simulink model "scheme_robust_control"  (R2025a)
settings: Solver=ode3  StartTime=0.0  StopTime=40  FixedStep=dt  RelTol=1e-3
values from neighbouring files (symbols this model uses):
  dt = 0.01    [Planning_Adaptive_LTV.m]
  initial_positions_rad = rawJointPositions(1, :)'    [manipulator_sim.m]
  map_scale = 0.5    [Planning_Adaptive_LTV.m]
  N = numel(theta_points_rad)    [create_LPV_linearizer.m]
  waypoints = pathObj.States(:, 1:2)    [Planning_Adaptive_LTV.m]
  x0 = zeros(10, 1)    [Planning_Adaptive_LTV.m]
undefined symbols (not defined in the file or in its folder): control_params, p, X, Y, Z
libraries: sm_lib x179, nesl_utility x28, fl_lib x3, robotmaniplib x2
(part 4 of 4)

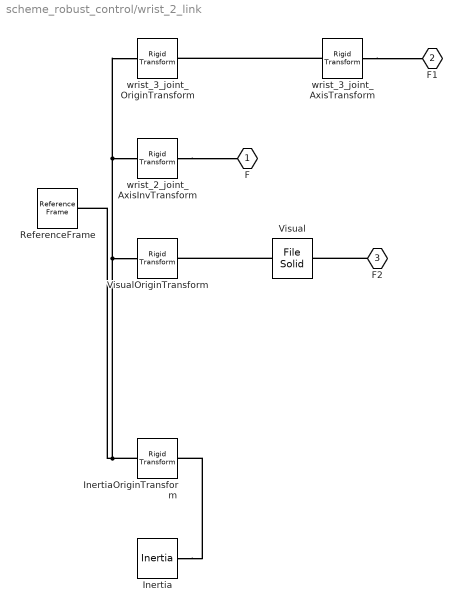
== system scheme_robust_control/wrist_2_link ==
  Inertia : sm_lib/Body Elements/Inertia  InertiaType=Custom  Mass=1.3  MassUnits=kg  CenterOfMass=[0, 0, 0]  CenterOfMassUnits=m  MomentsOfInertia=[0.00135617, 0.00096614, 0.00127827]  MomentsOfInertiaUnits=kg*m^2  ProductsOfInertia=[5.048000000000011e-05, 2.739999999999998e-06, 4.440000000000001e-06]  ProductsOfInertiaUnits=kg*m^2  GraphicType=None  MarkerShape=Inertia  MarkerSize=20  GraphicVisPropType=SimpleVisualProperties  GraphicDiffuseColor=[0.5 0.5 0.5]  GraphicOpacity=1  GraphicSpecularColor=[0.5 0.5 0.5 1.0]  GraphicAmbientColor=[0.15 0.15 0.15 1.0]  GraphicEmissiveColor=[0.0 0.0 0.0 1.0]  GraphicShininess=75
  InertiaOriginTransform : sm_lib/Frames and Transforms/Rigid Transform  RotationMethod=RotationSequence  FollAlignAxisA=+X  BaseAlignAxisA=+Y  FollAlignAxisB=+Y  BaseAlignAxisB=+Z  RotationStandardAxis=+Z  RotationAngle=0  RotationAngleUnits=deg  RotationArbitraryAxis=[0 0 1]  RotationSequenceAxes=BaseAxes  RotationSequence=XYZ  RotationSequenceAngles=[0, 0, 0]  RotationSequenceAnglesUnits=rad  RotationMatrix=[1 0 0;0 1 0;0 0 1]  Quaternion=[1 0 0 0]  TranslationMethod=Cartesian  TranslationCartesianOffset=[0, 0.01634, -0.0018]  TranslationCartesianOffsetUnits=m  TranslationStandardAxis=+Z  TranslationStandardOffset=0  TranslationStandardOffsetUnits=m  TranslationROffset=0  TranslationROffsetUnits=m  TranslationThetaOffset=0  TranslationThetaOffsetUnits=deg  TranslationZOffset=0  TranslationZOffsetUnits=m
  ReferenceFrame : sm_lib/Frames and Transforms/Reference Frame
  Visual : sm_lib/Body Elements/File Solid  ExtGeomFileName=C:\Users\chiar_zjcy1by\MATLAB Drive\FieldProject\generated\ros_packages\ur_description\meshes\ur5e\visual\wrist2.dae  UnitType=Custom  ExtGeomFileUnits=m  StepReaderType=HEX  ExportConvexHullGeometry=on  InertiaType=Custom  BasedOnType=DensityFromFile  Density=1000  DensityUnits=kg/m^3  Mass=0  MassUnits=kg  CenterOfMass=[0, 0, 0]  CenterOfMassUnits=m  MomentsOfInertia=[0, 0, 0]  MomentsOfInertiaUnits=kg*m^2  ProductsOfInertia=[0, 0, 0]  ProductsOfInertiaUnits=kg*m^2  GraphicType=FromGeometry  MarkerShape=Sphere  MarkerSize=10  GraphicVisPropType=SimpleVisualProperties  GraphicDiffuseColor=[0.5, 0.5, 0.5]  GraphicOpacity=1  GraphicSpecularColor=[0.5 0.5 0.5 1.0]  GraphicAmbientColor=[0.15 0.15 0.15 1.0]  GraphicEmissiveColor=[0.0 0.0 0.0 1.0]  GraphicShininess=75  DoExposeReferenceFrame=on  SerializedFrames=<Frames/>
  VisualOriginTransform : sm_lib/Frames and Transforms/Rigid Transform  RotationMethod=RotationSequence  FollAlignAxisA=+X  BaseAlignAxisA=+Y  FollAlignAxisB=+Y  BaseAlignAxisB=+Z  RotationStandardAxis=+Z  RotationAngle=0  RotationAngleUnits=deg  RotationArbitraryAxis=[0 0 1]  RotationSequenceAxes=BaseAxes  RotationSequence=XYZ  RotationSequenceAngles=[0, 0, 0]  RotationSequenceAnglesUnits=rad  RotationMatrix=[1 0 0;0 1 0;0 0 1]  Quaternion=[1 0 0 0]  TranslationMethod=Cartesian  TranslationCartesianOffset=[0, 0, -0.0997]  TranslationCartesianOffsetUnits=m  TranslationStandardAxis=+Z  TranslationStandardOffset=0  TranslationStandardOffsetUnits=m  TranslationROffset=0  TranslationROffsetUnits=m  TranslationThetaOffset=0  TranslationThetaOffsetUnits=deg  TranslationZOffset=0  TranslationZOffsetUnits=m
  wrist_2_joint_AxisInvTransform : sm_lib/Frames and Transforms/Rigid Transform  RotationMethod=ArbitraryAxis  FollAlignAxisA=+X  BaseAlignAxisA=+Y  FollAlignAxisB=+Y  BaseAlignAxisB=+Z  RotationStandardAxis=+Z  RotationAngle=0  RotationAngleUnits=rad  RotationArbitraryAxis=[1, 0, 0]  RotationSequenceAxes=FollowerAxes  RotationSequence=XYX  RotationSequenceAngles=[0 0 0]  RotationSequenceAnglesUnits=deg  RotationMatrix=[1 0 0;0 1 0;0 0 1]  Quaternion=[1 0 0 0]  TranslationMethod=Cartesian  TranslationCartesianOffset=[0, 0, 0]  TranslationCartesianOffsetUnits=m  TranslationStandardAxis=+Z  TranslationStandardOffset=0  TranslationStandardOffsetUnits=m  TranslationROffset=0  TranslationROffsetUnits=m  TranslationThetaOffset=0  TranslationThetaOffsetUnits=deg  TranslationZOffset=0  TranslationZOffsetUnits=m
  wrist_3_joint_AxisTransform : sm_lib/Frames and Transforms/Rigid Transform  RotationMethod=ArbitraryAxis  FollAlignAxisA=+X  BaseAlignAxisA=+Y  FollAlignAxisB=+Y  BaseAlignAxisB=+Z  RotationStandardAxis=+Z  RotationAngle=0  RotationAngleUnits=rad  RotationArbitraryAxis=[1, 0, 0]  RotationSequenceAxes=FollowerAxes  RotationSequence=XYX  RotationSequenceAngles=[0 0 0]  RotationSequenceAnglesUnits=deg  RotationMatrix=[1 0 0;0 1 0;0 0 1]  Quaternion=[1 0 0 0]  TranslationMethod=Cartesian  TranslationCartesianOffset=[0, 0, 0]  TranslationCartesianOffsetUnits=m  TranslationStandardAxis=+Z  TranslationStandardOffset=0  TranslationStandardOffsetUnits=m  TranslationROffset=0  TranslationROffsetUnits=m  TranslationThetaOffset=0  TranslationThetaOffsetUnits=deg  TranslationZOffset=0  TranslationZOffsetUnits=m
  wrist_3_joint_OriginTransform : sm_lib/Frames and Transforms/Rigid Transform  RotationMethod=RotationSequence  FollAlignAxisA=+X  BaseAlignAxisA=+Y  FollAlignAxisB=+Y  BaseAlignAxisB=+Z  RotationStandardAxis=+Z  RotationAngle=0  RotationAngleUnits=deg  RotationArbitraryAxis=[0 0 1]  RotationSequenceAxes=BaseAxes  RotationSequence=XYZ  RotationSequenceAngles=[-1.570796327, 1.224646799147353e-16, -1.224646799147353e-16]  RotationSequenceAnglesUnits=rad  RotationMatrix=[1 0 0;0 1 0;0 0 1]  Quaternion=[1 0 0 0]  TranslationMethod=Cartesian  TranslationCartesianOffset=[0, 0.09959999999999999, -2.042830148012698e-11]  TranslationCartesianOffsetUnits=m  TranslationStandardAxis=+Z  TranslationStandardOffset=0  TranslationStandardOffsetUnits=m  TranslationROffset=0  TranslationROffsetUnits=m  TranslationThetaOffset=0  TranslationThetaOffsetUnits=deg  TranslationZOffset=0  TranslationZOffsetUnits=m
  F : PMIOPort  Side=Left
  F1 : PMIOPort  Port=2  Side=Right
  F2 : PMIOPort  Port=3  Side=Left
  connections:
  Inertia/RConn1 -- InertiaOriginTransform/RConn1
  ReferenceFrame/RConn1 -- InertiaOriginTransform/LConn1 -- wrist_2_joint_AxisInvTransform/LConn1 -- wrist_3_joint_OriginTransform/LConn1 -- VisualOriginTransform/LConn1
  Visual/RConn1 -- VisualOriginTransform/RConn1
  wrist_2_joint_AxisInvTransform/RConn1 -- F/RConn1
  wrist_3_joint_AxisTransform/RConn1 -- F1/RConn1
  wrist_3_joint_AxisTransform/LConn1 -- wrist_3_joint_OriginTransform/RConn1
  F2/RConn1 -- Visual/LConn1

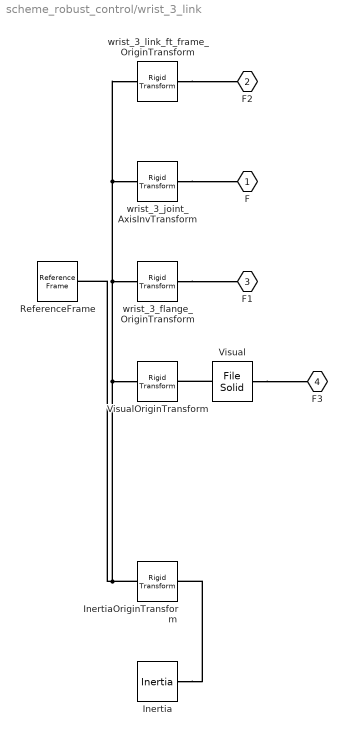
== system scheme_robust_control/wrist_3_link ==
  Inertia : sm_lib/Body Elements/Inertia  InertiaType=Custom  Mass=0.365  MassUnits=kg  CenterOfMass=[0, 0, 0]  CenterOfMassUnits=m  MomentsOfInertia=[0.00018694, 0.00018908, 0.00025756]  MomentsOfInertiaUnits=kg*m^2  ProductsOfInertia=[-9.2e-07, -1.7e-07, 5.999999999999999e-08]  ProductsOfInertiaUnits=kg*m^2  GraphicType=None  MarkerShape=Inertia  MarkerSize=20  GraphicVisPropType=SimpleVisualProperties  GraphicDiffuseColor=[0.5 0.5 0.5]  GraphicOpacity=1  GraphicSpecularColor=[0.5 0.5 0.5 1.0]  GraphicAmbientColor=[0.15 0.15 0.15 1.0]  GraphicEmissiveColor=[0.0 0.0 0.0 1.0]  GraphicShininess=75
  InertiaOriginTransform : sm_lib/Frames and Transforms/Rigid Transform  RotationMethod=RotationSequence  FollAlignAxisA=+X  BaseAlignAxisA=+Y  FollAlignAxisB=+Y  BaseAlignAxisB=+Z  RotationStandardAxis=+Z  RotationAngle=0  RotationAngleUnits=deg  RotationArbitraryAxis=[0 0 1]  RotationSequenceAxes=BaseAxes  RotationSequence=XYZ  RotationSequenceAngles=[0, 0, 0]  RotationSequenceAnglesUnits=rad  RotationMatrix=[1 0 0;0 1 0;0 0 1]  Quaternion=[1 0 0 0]  TranslationMethod=Cartesian  TranslationCartesianOffset=[0, 0, -0.001159]  TranslationCartesianOffsetUnits=m  TranslationStandardAxis=+Z  TranslationStandardOffset=0  TranslationStandardOffsetUnits=m  TranslationROffset=0  TranslationROffsetUnits=m  TranslationThetaOffset=0  TranslationThetaOffsetUnits=deg  TranslationZOffset=0  TranslationZOffsetUnits=m
  ReferenceFrame : sm_lib/Frames and Transforms/Reference Frame
  Visual : sm_lib/Body Elements/File Solid  ExtGeomFileName=C:\Users\chiar_zjcy1by\MATLAB Drive\FieldProject\generated\ros_packages\ur_description\meshes\ur5e\visual\wrist3.dae  UnitType=Custom  ExtGeomFileUnits=m  StepReaderType=HEX  ExportConvexHullGeometry=on  InertiaType=Custom  BasedOnType=DensityFromFile  Density=1000  DensityUnits=kg/m^3  Mass=0  MassUnits=kg  CenterOfMass=[0, 0, 0]  CenterOfMassUnits=m  MomentsOfInertia=[0, 0, 0]  MomentsOfInertiaUnits=kg*m^2  ProductsOfInertia=[0, 0, 0]  ProductsOfInertiaUnits=kg*m^2  GraphicType=FromGeometry  MarkerShape=Sphere  MarkerSize=10  GraphicVisPropType=SimpleVisualProperties  GraphicDiffuseColor=[0.5, 0.5, 0.5]  GraphicOpacity=1  GraphicSpecularColor=[0.5 0.5 0.5 1.0]  GraphicAmbientColor=[0.15 0.15 0.15 1.0]  GraphicEmissiveColor=[0.0 0.0 0.0 1.0]  GraphicShininess=75  DoExposeReferenceFrame=on  SerializedFrames=<Frames/>
  VisualOriginTransform : sm_lib/Frames and Transforms/Rigid Transform  RotationMethod=RotationSequence  FollAlignAxisA=+X  BaseAlignAxisA=+Y  FollAlignAxisB=+Y  BaseAlignAxisB=+Z  RotationStandardAxis=+Z  RotationAngle=0  RotationAngleUnits=deg  RotationArbitraryAxis=[0 0 1]  RotationSequenceAxes=BaseAxes  RotationSequence=XYZ  RotationSequenceAngles=[1.570796326794897, 0, 0]  RotationSequenceAnglesUnits=rad  RotationMatrix=[1 0 0;0 1 0;0 0 1]  Quaternion=[1 0 0 0]  TranslationMethod=Cartesian  TranslationCartesianOffset=[0, 0, -0.0989]  TranslationCartesianOffsetUnits=m  TranslationStandardAxis=+Z  TranslationStandardOffset=0  TranslationStandardOffsetUnits=m  TranslationROffset=0  TranslationROffsetUnits=m  TranslationThetaOffset=0  TranslationThetaOffsetUnits=deg  TranslationZOffset=0  TranslationZOffsetUnits=m
  wrist_3_flange_OriginTransform : sm_lib/Frames and Transforms/Rigid Transform  RotationMethod=RotationSequence  FollAlignAxisA=+X  BaseAlignAxisA=+Y  FollAlignAxisB=+Y  BaseAlignAxisB=+Z  RotationStandardAxis=+Z  RotationAngle=0  RotationAngleUnits=deg  RotationArbitraryAxis=[0 0 1]  RotationSequenceAxes=BaseAxes  RotationSequence=XYZ  RotationSequenceAngles=[-1.570796326794897, -1.570796326794897, 0]  RotationSequenceAnglesUnits=rad  RotationMatrix=[1 0 0;0 1 0;0 0 1]  Quaternion=[1 0 0 0]  TranslationMethod=Cartesian  TranslationCartesianOffset=[0, 0, 0]  TranslationCartesianOffsetUnits=m  TranslationStandardAxis=+Z  TranslationStandardOffset=0  TranslationStandardOffsetUnits=m  TranslationROffset=0  TranslationROffsetUnits=m  TranslationThetaOffset=0  TranslationThetaOffsetUnits=deg  TranslationZOffset=0  TranslationZOffsetUnits=m
  wrist_3_joint_AxisInvTransform : sm_lib/Frames and Transforms/Rigid Transform  RotationMethod=ArbitraryAxis  FollAlignAxisA=+X  BaseAlignAxisA=+Y  FollAlignAxisB=+Y  BaseAlignAxisB=+Z  RotationStandardAxis=+Z  RotationAngle=0  RotationAngleUnits=rad  RotationArbitraryAxis=[1, 0, 0]  RotationSequenceAxes=FollowerAxes  RotationSequence=XYX  RotationSequenceAngles=[0 0 0]  RotationSequenceAnglesUnits=deg  RotationMatrix=[1 0 0;0 1 0;0 0 1]  Quaternion=[1 0 0 0]  TranslationMethod=Cartesian  TranslationCartesianOffset=[0, 0, 0]  TranslationCartesianOffsetUnits=m  TranslationStandardAxis=+Z  TranslationStandardOffset=0  TranslationStandardOffsetUnits=m  TranslationROffset=0  TranslationROffsetUnits=m  TranslationThetaOffset=0  TranslationThetaOffsetUnits=deg  TranslationZOffset=0  TranslationZOffsetUnits=m
  wrist_3_link_ft_frame_OriginTransform : sm_lib/Frames and Transforms/Rigid Transform  RotationMethod=RotationSequence  FollAlignAxisA=+X  BaseAlignAxisA=+Y  FollAlignAxisB=+Y  BaseAlignAxisB=+Z  RotationStandardAxis=+Z  RotationAngle=0  RotationAngleUnits=deg  RotationArbitraryAxis=[0 0 1]  RotationSequenceAxes=BaseAxes  RotationSequence=XYZ  RotationSequenceAngles=[3.141592653589793, -0, 0]  RotationSequenceAnglesUnits=rad  RotationMatrix=[1 0 0;0 1 0;0 0 1]  Quaternion=[1 0 0 0]  TranslationMethod=Cartesian  TranslationCartesianOffset=[0, 0, 0]  TranslationCartesianOffsetUnits=m  TranslationStandardAxis=+Z  TranslationStandardOffset=0  TranslationStandardOffsetUnits=m  TranslationROffset=0  TranslationROffsetUnits=m  TranslationThetaOffset=0  TranslationThetaOffsetUnits=deg  TranslationZOffset=0  TranslationZOffsetUnits=m
  F : PMIOPort  Side=Left
  F2 : PMIOPort  Port=2  Side=Right
  F1 : PMIOPort  Port=3  Side=Right
  F3 : PMIOPort  Port=4  Side=Left
  connections:
  Inertia/RConn1 -- InertiaOriginTransform/RConn1
  ReferenceFrame/RConn1 -- InertiaOriginTransform/LConn1 -- wrist_3_joint_AxisInvTransform/LConn1 -- wrist_3_link_ft_frame_OriginTransform/LConn1 -- wrist_3_flange_OriginTransform/LConn1 -- VisualOriginTransform/LConn1
  Visual/RConn1 -- VisualOriginTransform/RConn1
  wrist_3_flange_OriginTransform/RConn1 -- F1/RConn1
  wrist_3_joint_AxisInvTransform/RConn1 -- F/RConn1
  wrist_3_link_ft_frame_OriginTransform/RConn1 -- F2/RConn1
  Visual/LConn1 -- F3/RConn1

== matlab function scheme_robust_control/MATLAB Function ==
  data: D input; Q input; eps input; rho input; errdata input; w output
function w = compute_w(D,Q,eps,rho,errdata)
e = errdata(1:6);
e_dot = errdata(7:12);

csi = [e; e_dot];

z = D'*Q*csi;

if (norm(z) > eps)
    w = (rho*z)/norm(z);
else
    w = (rho*z)/eps;
end

end

== matlab function scheme_robust_control/NL controller ==
  settings: updateMethod=DISCRETE
  data: x input; tau output; waypoints input; p parameter; control_params parameter; map_scale parameter; dt parameter; tau_ey output; tau_ex output
function [tau,tau_ey,tau_ex] = fcn(x, waypoints, p, control_params, map_scale,dt)
% This function implements the full cascaded controller inside a 
% single Simulink MATLAB Function block.

% persistent variables hold their values between simulation steps.
% This is how we keep track of the current waypoint and integral error.
persistent current_waypoint_idx;
persistent integral_error;

% Initialize persistent variables on the first run
if isempty(current_waypoint_idx)
    current_waypoint_idx = 1;
    integral_error = zeros(2,1); % [integral_error_x; integral_error_y]
end

% --- Waypoint Manager ---
waypoint_reach_threshold = 0.15 * map_scale;
p_target = waypoints(current_waypoint_idx, :)';

p_current = [p.r_S * x(5); -p.r_S * x(4)];
distance_to_target = norm(p_current - p_target);

if (distance_to_target < waypoint_reach_threshold) && (current_waypoint_idx < size(waypoints, 1))
    current_waypoint_idx = current_waypoint_idx + 1;
end

% --- Controller Logic (adapted from your script) ---
% Unpack controller parameters
K = control_params.K;
A = control_params.A_lqr;
B = control_params.B_lqr;
Kp_pos = control_params.Kp_pos;
Kp_inner = control_params.Kp_inner;
Ki_inner = control_params.Ki_inner;

% Unpack states
theta_x = x(1); dot_theta_x = x(6);
theta_y = x(2); dot_theta_y = x(7);
phi_x   = x(4); dot_phi_x   = x(9);
phi_y   = x(5); dot_phi_y   = x(10);

% Note: We now manage the integral error inside this function
int_err_vx = integral_error(1);
int_err_vy = integral_error(2);

% --- STEP 1: OUTER-MOST LOOP (P Position Controller) ---
error_pos = p_target - p_current;
v_cmd = Kp_pos * error_pos;
dot_phi_cmd_y = v_cmd(1) / p.r_S;
dot_phi_cmd_x = -v_cmd(2) / p.r_S;

% -- Sagittal Plane (Y) --
state_y = [theta_y; phi_y; dot_theta_y; dot_phi_y];
command_state_y = [0; phi_y; 0; dot_phi_cmd_y];
%LQR
tau_ry = -K * (state_y - command_state_y);

% -- Frontal Plane (X) --
state_x = [theta_x; phi_x; dot_theta_x; dot_phi_x];
command_state_x = [0; phi_x; 0; dot_phi_cmd_x];
%LQR
tau_rx = -K * (state_x - command_state_x);
% --- ASSEMBLY ---
tau_z = 0; 
tau_r = [tau_rx; tau_ry; tau_z];
dx = stateDerivative3D_generated(x(1:10),p, tau_r);
dot_phi_rx =dx(4);
dot_phi_ry=dx(5);

speed_error_x = dot_phi_rx - dot_phi_x;
tau_ex = Kp_inner * speed_error_x + Ki_inner * int_err_vx;
tau_x = tau_rx + tau_ex;

speed_error_y = dot_phi_ry - dot_phi_y;
%PI
tau_ey = Kp_inner * speed_error_y + Ki_inner * int_err_vy;
tau_y = tau_ry + tau_ey;

% --- FINAL ASSEMBLY ---
tau_z = 0; 
tau = [tau_x; tau_y; tau_z];
% --- Update Integral for next time step ---
integral_error = integral_error + [speed_error_x; speed_error_y] * dt;



end

function dx = stateDerivative3D_generated(x, p, tau)
    % SW was assumed to not spin relative to the ground
    
    % Unpack state vector (10 elements)
    theta_x = x(1); dot_theta_x = x(6);
    theta_y = x(2); dot_theta_y = x(7);
    theta_z = x(3); dot_theta_z = x(8);
    % phi_x   = x(4); % Not needed for dynamics
    % phi_y   = x(5); % Not needed for dynamics
    dot_phi_x   = x(9);
    dot_phi_y   = x(10);
    
    % Unpack input torques
    tau_x = tau(1);
    tau_y = tau(2);
    tau_z = tau(3);

    % --- Prepare arguments for auto-generated functions ---
    % Argument list for parameters (order MUST match the generator script)
    params_arg = [p.m_U, p.I_Uy, p.I_Ux, p.l_U, p.m_S, p.I_S, p.r_S, p.g, p.b_theta, p.b_phi];

    % --- X-Z Plane (Roll) Dynamics ---
    states_arg_x = [theta_x, dot_theta_x, dot_phi_x];
    inputs_arg_x = [tau_x];
    ddot_theta_x = autogen_ddot_theta_x(states_arg_x, inputs_arg_x, params_arg);
    ddot_phi_x   = autogen_ddot_phi_x(states_arg_x, inputs_arg_x, params_arg);

    % --- Y-Z Plane (Pitch) Dynamics ---
    states_arg_y = [theta_y, dot_theta_y, dot_phi_y];
    inputs_arg_y = [tau_y];
    ddot_theta_y = autogen_ddot_theta_y(states_arg_y, inputs_arg_y, params_arg);
    ddot_phi_y   = autogen_ddot_phi_y(states_arg_y, inputs_arg_y, params_arg);
    
    % --- Transversal Plane Dynamics (Yaw) ---
    % Using the simple decoupled model from your original script
    ddot_theta_z = (tau_z - p.fz * dot_theta_z) / p.Iz;
    
    % --- Assemble the state derivative vector dx ---
    dx = [
        dot_theta_x;    % dx(1) = d(theta_x)/dt
        dot_theta_y;    % dx(2) = d(theta_y)/dt
        dot_theta_z;    % dx(3) = d(theta_z)/dt
        dot_phi_x;      % dx(4) = d(phi_x)/dt
        dot_phi_y;      % dx(5) = d(phi_y)/dt
        ddot_theta_x;   % dx(6) = d(dot_theta_x)/dt
        ddot_theta_y;   % dx(7) = d(dot_theta_y)/dt
        ddot_theta_z;   % dx(8) = d(dot_theta_z)/dt
        ddot_phi_x;     % dx(9) = d(dot_phi_x)/dt
        ddot_phi_y;     % dx(10)= d(dot_phi_y)/dt
    ];
end

== matlab function scheme_robust_control/BallBot Plant1/MATLAB Function ==
  data: dx output; x input; p parameter; tau input; wrench_ext input
function dx = stateDerivative3D_with_exforce(x, p, tau, wrench_ext)
    % MODIFICATION 1: The function now accepts a 4th argument, 'wrench_ext',
    % which is a vector containing the external forces and torques from Simulink.
    
    % Unpack state vector (10 elements)
    theta_x = x(1); dot_theta_x = x(6);
    theta_y = x(2); dot_theta_y = x(7);
    theta_z = x(3); dot_theta_z = x(8);
    % phi_x   = x(4); % Not needed for dynamics
    % phi_y   = x(5); % Not needed for dynamics
    dot_phi_x   = x(9);
    dot_phi_y   = x(10);
    
    % Unpack input torques
    tau_x = tau(1);
    tau_y = tau(2);
    tau_z = tau(3);

     % Unpack the external wrench vector from the new input ---
    % Expected order: [F_px, F_py, F_pz, tau_px, tau_py]
    F_px   = wrench_ext(1);
    F_py   = wrench_ext(2);
    F_pz   = wrench_ext(3);
    tau_px = wrench_ext(4);
    tau_py = wrench_ext(5);

    % --- Prepare arguments for auto-generated functions ---
    % Create separate parameter vectors for each plane, now including h_app
    % Note: I_Ux is for roll, I_Uy is for pitch.
    params_arg_roll = [p.m_U, p.I_Ux, p.l_U, p.m_S, p.I_S, p.r_S, p.g, p.b_phi, p.h_app];
    params_arg_pitch = [p.m_U, p.I_Uy, p.l_U, p.m_S, p.I_S, p.r_S, p.g, p.b_phi, p.h_app];
    
    external_vars_x = [F_py, F_pz, tau_px]; % For Roll dynamics
    external_vars_y = [F_px, F_pz, tau_py]; % For Pitch dynamics

    % --- X-Z Plane (Roll) Dynamics ---
    states_arg_x = [theta_x, dot_theta_x, dot_phi_x];
    inputs_arg_x = [tau_x];
    ddot_theta_x = autogen_ddot_theta_x_exforce(states_arg_x, inputs_arg_x, params_arg_roll, external_vars_x);
    ddot_phi_x   = autogen_ddot_phi_x_exforce(states_arg_x, inputs_arg_x, params_arg_roll, external_vars_x);
    

    % --- Y-Z Plane (Pitch) Dynamics ---
    states_arg_y = [theta_y, dot_theta_y, dot_phi_y];
    inputs_arg_y = [tau_y];
    ddot_theta_y = autogen_ddot_theta_y_exforce(states_arg_y, inputs_arg_y, params_arg_pitch, external_vars_y);
    ddot_phi_y   = autogen_ddot_phi_y_exforce(states_arg_y, inputs_arg_y, params_arg_pitch, external_vars_y);
    
    % --- Transversal Plane Dynamics (Yaw) ---
    % external forces at the center of the top surface are assumed not to produce yaw torque.
    ddot_theta_z = (tau_z - p.fz * dot_theta_z) / p.Iz;
    
    % --- Assemble the state derivative vector dx ---
    dx = [
        dot_theta_x;    % dx(1) = d(theta_x)/dt
        dot_theta_y;    % dx(2) = d(theta_y)/dt
        dot_theta_z;    % dx(3) = d(theta_z)/dt
        dot_phi_x;      % dx(4) = d(phi_x)/dt
        dot_phi_y;      % dx(5) = d(phi_y)/dt
        ddot_theta_x;   % dx(6) = d(dot_theta_x)/dt
        ddot_theta_y;   % dx(7) = d(dot_theta_y)/dt
        ddot_theta_z;   % dx(8) = d(dot_theta_z)/dt
        ddot_phi_x;     % dx(9) = d(dot_phi_x)/dt
        ddot_phi_y;     % dx(10)= d(dot_phi_y)/dt
    ];
end
